simulink model "radar_noise"  (R2016b)
settings: Solver=VariableStepAuto  StartTime=0.0  StopTime=10.0  RelTol=1e-3
values from neighbouring files (symbols this model uses):
  K = gain(x)    [radar_sweep.m]    (also in sweep.m; sweep_1.m; sweep_2.m; wind_sweep.m)
settings Model: Creator=ammar_laptop  LastModifiedBy=ammar_laptop

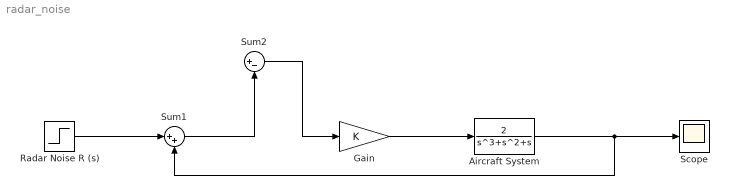
== system radar_noise ==
  "Aircraft System " : TransferFcn  Numerator=[2]  Denominator=[1 1 1 0]
  Gain : Gain  Gain=K
  Radar Noise R (s) : Step  SampleTime=0
  Scope : Scope
  Sum1 : Sum  Inputs=|++
  Sum2 : Sum  Inputs=|+-
  wires:
  Gain/1 -> "Aircraft System "/1
  Sum2/1 -> Gain/1
  Sum1/1 -> Sum2/2
  Radar Noise R (s)/1 -> Sum1/1
  "Aircraft System "/1 -> Sum1/2, Scope/1
